simulink model "RC_simple"  (R2018b)
settings: Solver=VariableStepAuto  StartTime=0.0  StopTime=10.0  RelTol=1e-3
model workspace (MATLAB code in the model file):
  | C = 1e-3; % F
  | R = 1e3; % Ohm
settings Model: Creator=kjartan  LastModifiedBy=kjartan

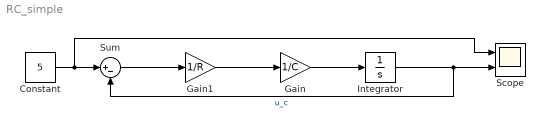
== system RC_simple ==
  Constant : Constant  Value=5
  Gain : Gain  Gain=1/C
  Gain1 : Gain  Gain=1/R
  Integrator : Integrator
  Scope : Scope  NumInputPorts=2
  Sum : Sum  Inputs=|+-
  wires:
  Integrator/1 -> Sum/2, Scope/2  "u_c"
  Gain/1 -> Integrator/1
  Gain1/1 -> Gain/1
  Constant/1 -> Scope/1, Sum/1
  Sum/1 -> Gain1/1
